simulink model "MMFA"  (R2020b)
settings: Solver=VariableStepAuto  StartTime=0.0  StopTime=22  RelTol=1e-3
libraries: dspvision x5, commanapbnd3 x3, dsparch4 x1
settings Model: Creator=fernando  LastModifiedBy=fernando

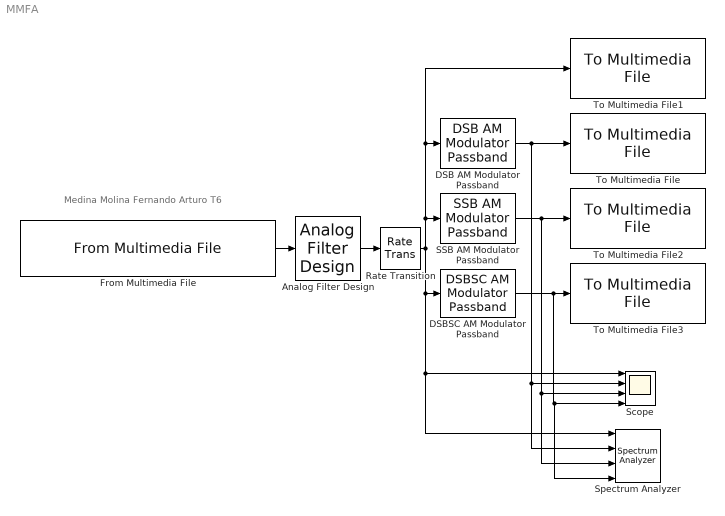
== system MMFA ==
  note: Medina Molina Fernando Arturo T6
  Analog Filter Design : dsparch4/Analog Filter Design  method=Butterworth  filttype=Lowpass  N=8  Wlo=2*pi*4e3  Whi=80  Rp=2  Rs=40
  DSB AM Modulator Passband : commanapbnd3/DSB AM Modulator Passband  Fc=10e3  Ph=0  Offset=1
      settings: SourceProductBaseCode=CM
  DSBSC AM Modulator Passband : commanapbnd3/DSBSC AM Modulator Passband  Fc=300  Ph=0
      settings: SourceProductBaseCode=CM
  From Multimedia File : dspvision/From Multimedia File  inputFilename=/home/fernando/Documentos/Sistemas de comunicaciones/Clases/Tarea 6/WhatsApp Ptt 2020-12-02 at 18.26.42.ogg  readRange=[1 Inf]  loop=on  numPlays=inf  outputStreams=Audio only  videoDataType=single  audioDataType=double  inheritSampleTime=on  userDefinedSampleTime=1/30  noAudioOutput=off  isIntensityVideo=off  fourcc=RGB  colorVideoFormat=Separate color signals  outputEOF=off  dataOrg=Column-major  audioFrameSize=1  computeAudioFrameSize=off  outSamplingMode=Sample based
  Rate Transition : RateTransition  OutPortSampleTime=1/44100/2
  SSB AM Modulator Passband : commanapbnd3/SSB AM Modulator Passband  Fc=300  Ph=0  Sd=Upper  Ho=100
      settings: SourceProductBaseCode=CM
  Scope : Scope  NumInputPorts=4
  Spectrum Analyzer : SpectrumAnalyzer  NumInputPorts=4
  To Multimedia File : dspvision/To Multimedia File  outputFilename=/home/fernando/Documentos/Sistemas de comunicaciones/Clases/Tarea 6/SalidaDSB.wav  streamSelection=Audio only  videoCompressor=None (uncompressed)  audioCompressor=None (uncompressed)  imagePorts=Separate color signals  fileType=WAV  audioDatatype=16-bit integer  fourcc=RGB  videoQuality=75  mj2000CompFactor=10
  To Multimedia File1 : dspvision/To Multimedia File  outputFilename=/home/fernando/Documentos/Sistemas de comunicaciones/Clases/Tarea 6/SalidaFiltro.wav  streamSelection=Audio only  videoCompressor=None (uncompressed)  audioCompressor=None (uncompressed)  imagePorts=Separate color signals  fileType=WAV  audioDatatype=16-bit integer  fourcc=RGB  videoQuality=75  mj2000CompFactor=10
  To Multimedia File2 : dspvision/To Multimedia File  outputFilename=/home/fernando/Documentos/Sistemas de comunicaciones/Clases/Tarea 6/SalidaSSB.wav  streamSelection=Audio only  videoCompressor=None (uncompressed)  audioCompressor=None (uncompressed)  imagePorts=Separate color signals  fileType=WAV  audioDatatype=16-bit integer  fourcc=RGB  videoQuality=75  mj2000CompFactor=10
  To Multimedia File3 : dspvision/To Multimedia File  outputFilename=/home/fernando/Documentos/Sistemas de comunicaciones/Clases/Tarea 6/SalidaDSBSC.wav  streamSelection=Audio only  videoCompressor=None (uncompressed)  audioCompressor=None (uncompressed)  imagePorts=Separate color signals  fileType=WAV  audioDatatype=16-bit integer  fourcc=RGB  videoQuality=75  mj2000CompFactor=10
  wires:
  From Multimedia File/1 -> Analog Filter Design/1
  Analog Filter Design/1 -> Rate Transition/1
  Rate Transition/1 -> To Multimedia File1/1, DSB AM Modulator Passband/1, SSB AM Modulator Passband/1, Scope/1, Spectrum Analyzer/1, DSBSC AM Modulator Passband/1
  DSB AM Modulator Passband/1 -> Spectrum Analyzer/2, Scope/2, To Multimedia File/1
  SSB AM Modulator Passband/1 -> Scope/3, Spectrum Analyzer/3, To Multimedia File2/1
  DSBSC AM Modulator Passband/1 -> Spectrum Analyzer/4, Scope/4, To Multimedia File3/1
